simulink model "Path_planner_with_controller_localization"  (R2017b)
settings: Solver=FixedStepDiscrete  StartTime=0.0  StopTime=t  FixedStep=dt  RelTol=1e-3
values from neighbouring files (symbols this model uses):
  d = 0.15    [extendedKalman.m]    (also in extendedKalmanFilter.m; plant.m = 0.24; runV3.m; runpathfollower.m)
  dt = 0.1    [extendedKalmanFilter.m]    (also in matlab.mat; runV3.m; rungen.m; runpathfollower.m)
  k1 = 8    [runpathfollower.m]    (also in runpathplanner.m = 1)
  k2 = 1    [runpathfollower.m]    (also in runpathplanner.m)
  pl = 4    [runpathfollower.m]    (also in runpathplanner.m = 10)
  pr = 1    [runpathfollower.m]
  pthetai = 45*pi/180    (= 0.785398163397)    [runpathfollower.m]    (also in runpathplanner.m)
  pxi = 2    [runpathfollower.m]    (also in runpathplanner.m = 0)
  pyi = 2    [runpathfollower.m]    (also in runpathplanner.m)
  velocity = 0.3    [runpathfollower.m]    (also in runpathplanner.m)
  xi0 = [0 0 0 0 0 0 0 0]    [matlab.mat]    (also in runV3.m = [0 0 0 0 0 0 0 0]'; runpathfollower.m = [xi,yi,0,0,0,0,theta_mi,0]'; runpathplanner.m = [xi,yi,0,0,0,0,theta_mi,0]')
libraries: simulink x10
settings Model: Creator=nisha  LastModifiedBy=nisha

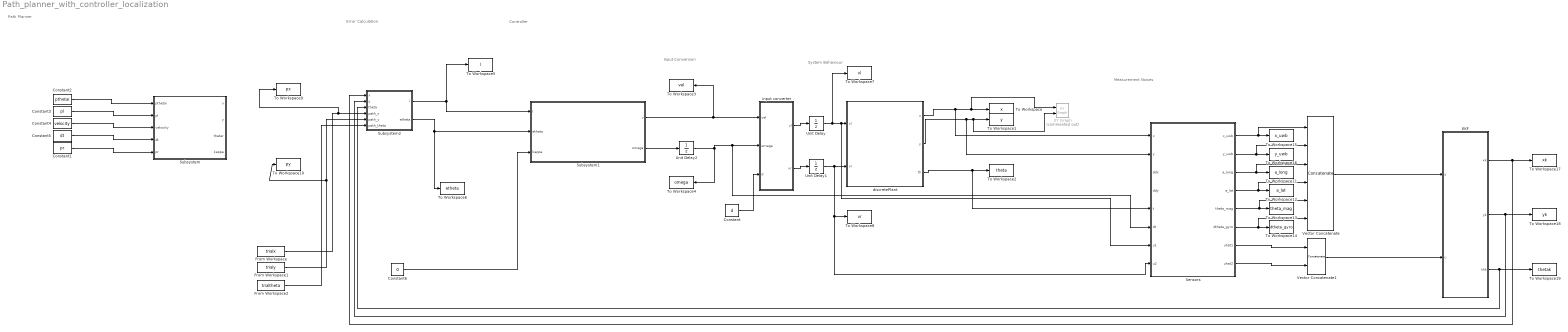
== system Path_planner_with_controller_localization ==
  note: Controller
  note: Error Calculation
  note: Measurement Noises
  note: System Behaviour
  note: Input Conversion
  note: Path Planner
  Constant : Constant  Value=d
  Constant1 : Constant  Value=pr
  Constant2 : Constant  Value=pthetai
  Constant3 : Constant  Value=pl
  Constant4 : Constant  Value=velocity
  Constant5 : Constant  Value=dt
  Constant6 : Constant  Value=0
  EKF : Subsystem
  From Workspace : FromWorkspace  VariableName=trialx
  From Workspace1 : FromWorkspace  VariableName=trialy
  From Workspace2 : FromWorkspace  VariableName=trialtheta
  Sensors : Subsystem  Description=dfg
  Subsystem : Subsystem
  Subsystem1 : Subsystem
  Subsystem2 : Subsystem
  To Workspace : ToWorkspace  VariableName=x  SampleTime=-1
  To Workspace1 : ToWorkspace  VariableName=y  SampleTime=-1
  To Workspace10 : ToWorkspace  VariableName=py  SampleTime=-1
  To Workspace11 : ToWorkspace  VariableName=a_long  SampleTime=-1
  To Workspace12 : ToWorkspace  VariableName=a_lat  SampleTime=-1
  To Workspace13 : ToWorkspace  VariableName=theta_mag  SampleTime=-1
  To Workspace14 : ToWorkspace  VariableName=dtheta_gyro  SampleTime=-1
  To Workspace15 : ToWorkspace  VariableName=x_uwb  SampleTime=-1
  To Workspace16 : ToWorkspace  VariableName=y_uwb  SampleTime=-1
  To Workspace17 : ToWorkspace  VariableName=xk  SampleTime=-1
  To Workspace18 : ToWorkspace  VariableName=yk  SampleTime=-1
  To Workspace19 : ToWorkspace  VariableName=thetak  SampleTime=-1
  To Workspace2 : ToWorkspace  VariableName=theta  SampleTime=-1
  To Workspace3 : ToWorkspace  VariableName=vel  SampleTime=-1
  To Workspace4 : ToWorkspace  VariableName=omega  SampleTime=-1
  To Workspace5 : ToWorkspace  VariableName=l  SampleTime=-1
  To Workspace6 : ToWorkspace  VariableName=etheta  SampleTime=-1
  To Workspace7 : ToWorkspace  VariableName=vl  SampleTime=-1
  To Workspace8 : ToWorkspace  VariableName=vr  SampleTime=-1
  To Workspace9 : ToWorkspace  VariableName=px  SampleTime=-1
  Unit Delay : UnitDelay  SampleTime=-1
  Unit Delay1 : UnitDelay  SampleTime=-1
  Unit Delay2 : UnitDelay  SampleTime=-1
  Vector Concatenate : Concatenate  NumInputs=6
  Vector Concatenate1 : Concatenate
  XY Graph : simulink/Sinks/XY Graph  Commented=on  xmin=0  xmax=10  ymin=2  ymax=12  st=-1
  discretePlant : Subsystem
  input converter : MATLAB Function  TreatAsAtomicUnit=on
  wires:
  Constant4/1 -> Subsystem/3(velocity)
  Constant3/1 -> Subsystem/2(pl)
  Constant2/1 -> Subsystem/1(pthetai)
  Constant5/1 -> Subsystem/4(dt)
  discretePlant/3(th) -> Sensors/5(t), To Workspace2/1
  Subsystem2/1(l) -> Subsystem1/1(l), To Workspace5/1
  Subsystem2/2(etheta) -> To Workspace6/1, Subsystem1/2(etheta)
  input converter/2(vr) -> Unit Delay1/1
  discretePlant/1(x) -> Sensors/1(x), XY Graph/1, To Workspace/1
  Constant/1 -> input converter/3(d)
  Subsystem1/1(v) -> To Workspace3/1, input converter/1(vel)
  Unit Delay/1 -> To Workspace7/1, Sensors/7(u1), discretePlant/1(vl)
  discretePlant/2(y) -> Sensors/2(y), XY Graph/2, To Workspace1/1
  input converter/1(vl) -> Unit Delay/1
  Subsystem1/2(omega) -> Unit Delay2/1
  Constant1/1 -> Subsystem/5(pr)
  Sensors/6(dtheta_gyro) -> To Workspace14/1, Vector Concatenate/6
  Sensors/8(uhat2) -> Vector Concatenate1/2
  Vector Concatenate1/1 -> EKF/2(u)
  Sensors/7(uhat1) -> Vector Concatenate1/1
  Sensors/3(a_long) -> Vector Concatenate/3, To Workspace11/1
  Sensors/5(theta_mag) -> Vector Concatenate/5, To Workspace13/1
  EKF/1(xk) -> To Workspace17/1, Subsystem2/1(x)
  Sensors/4(a_lat) -> Vector Concatenate/4, To Workspace12/1
  Sensors/1("x_uwb ") -> Vector Concatenate/1, To Workspace15/1
  Vector Concatenate/1 -> EKF/1(y)
  Sensors/2(y_uwb) -> Vector Concatenate/2, To Workspace16/1
  Unit Delay1/1 -> To Workspace8/1, Sensors/8(u2), discretePlant/2(vr)
  EKF/2(yk) -> To Workspace18/1, Subsystem2/2(y)
  EKF/3(thk) -> To Workspace19/1, Subsystem2/3(theta)
  Unit Delay2/1 -> Sensors/6(dt), input converter/2(omega), To Workspace4/1
  Constant6/1 -> Subsystem1/3(kappa)
  From Workspace/1 -> To Workspace9/1, Subsystem2/4(path_x)
  From Workspace1/1 -> To Workspace10/1, Subsystem2/5(path_y)
  From Workspace2/1 -> Subsystem2/6(path_theta)

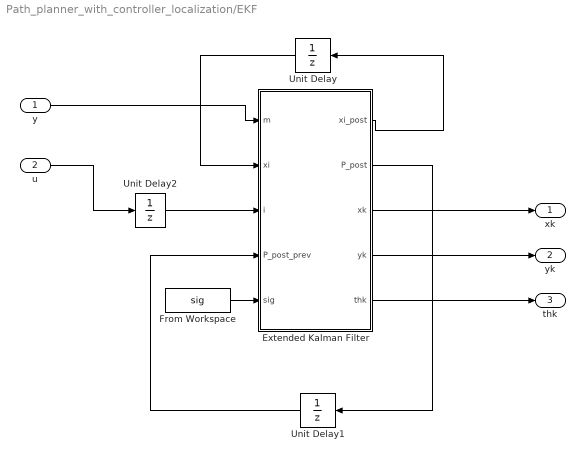
== system Path_planner_with_controller_localization/EKF ==
  y : Inport
  u : Inport  Port=2
  Extended Kalman Filter : MATLAB Function  TreatAsAtomicUnit=on
  From Workspace : FromWorkspace  VariableName=sig  SampleTime=0
  Unit Delay : UnitDelay  InitialCondition=xi0  SampleTime=-1
  Unit Delay1 : UnitDelay  InitialCondition=zeros(8,8)  SampleTime=-1
  Unit Delay2 : UnitDelay  InitialCondition=[0;0]  SampleTime=-1
  xk : Outport
  yk : Outport  Port=2
  thk : Outport  Port=3
  wires:
  Extended Kalman Filter/1(xi_post) -> Unit Delay/1
  y/1 -> Extended Kalman Filter/1(m)
  u/1 -> Unit Delay2/1
  Unit Delay2/1 -> Extended Kalman Filter/3(i)
  Unit Delay/1 -> Extended Kalman Filter/2(xi)
  Extended Kalman Filter/2(P_post) -> Unit Delay1/1
  Unit Delay1/1 -> Extended Kalman Filter/4(P_post_prev)
  Extended Kalman Filter/3(xk) -> xk/1
  Extended Kalman Filter/4(yk) -> yk/1
  From Workspace/1 -> Extended Kalman Filter/5(sig)
  Extended Kalman Filter/5(thk) -> thk/1

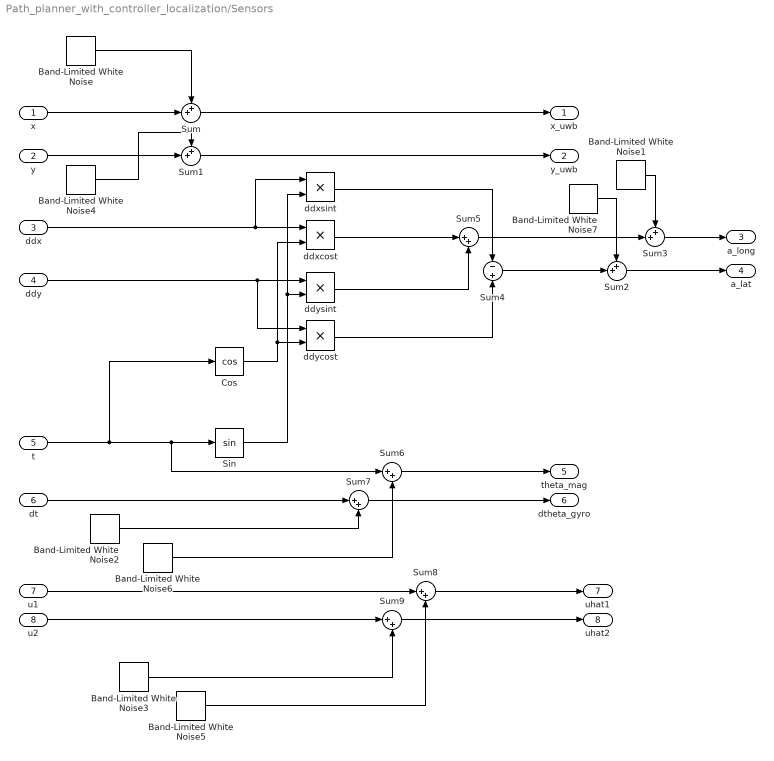
== system Path_planner_with_controller_localization/Sensors ==
  x : Inport
  y : Inport  Port=2
  ddx : Inport  Port=3
  ddy : Inport  Port=4
  t : Inport  Port=5
  dt : Inport  Port=6
  u1 : Inport  Port=7
  u2 : Inport  Port=8
  Band-Limited White Noise : simulink/Sources/Band-Limited White Noise  Cov=noiseUWB  Ts=dt  seed=[23341]
  Band-Limited White Noise1 : simulink/Sources/Band-Limited White Noise  Cov=noiseAcc  Ts=dt  seed=[23341]
  Band-Limited White Noise2 : simulink/Sources/Band-Limited White Noise  Cov=noiseGyro  Ts=dt  seed=[23341]
  Band-Limited White Noise3 : simulink/Sources/Band-Limited White Noise  Cov=noiseIn  Ts=dt  seed=[23341]
  Band-Limited White Noise4 : simulink/Sources/Band-Limited White Noise  Cov=noiseUWB  Ts=dt  seed=[23241]
  Band-Limited White Noise5 : simulink/Sources/Band-Limited White Noise  Cov=noiseIn  Ts=dt  seed=[23341]
  Band-Limited White Noise6 : simulink/Sources/Band-Limited White Noise  Cov=noiseMag  Ts=dt  seed=[23341]
  Band-Limited White Noise7 : simulink/Sources/Band-Limited White Noise  Cov=noiseAcc  Ts=dt  seed=[23341]
  Cos : Trigonometry  Operator=cos
  Sin : Trigonometry
  Sum{,1..3} (4 alike) : Sum  Inputs=++|
  Sum4 : Sum  Inputs=-|+
  Sum{5..9} (5 alike) : Sum  Inputs=|++
  ddxcost : Product
  ddxsint : Product
  ddycost : Product
  ddysint : Product
  "x_uwb " : Outport
  y_uwb : Outport  Port=2
  a_long : Outport  Port=3
  a_lat : Outport  Port=4
  theta_mag : Outport  Port=5
  dtheta_gyro : Outport  Port=6
  uhat1 : Outport  Port=7
  uhat2 : Outport  Port=8
  wires:
  x/1 -> Sum/2
  y/1 -> Sum1/2
  Band-Limited White Noise/1 -> Sum/1
  Sum/1 -> "x_uwb "/1
  Sum1/1 -> y_uwb/1
  Band-Limited White Noise1/1 -> Sum3/1
  t/1 -> Sum6/1, Sin/1, Cos/1
  ddx/1 -> ddxcost/1, ddxsint/1
  Cos/1 -> ddxcost/2, ddycost/2
  Sin/1 -> ddxsint/2, ddysint/2
  ddy/1 -> ddycost/1, ddysint/1
  Sum5/1 -> Sum3/2
  Sum4/1 -> Sum2/2
  ddxcost/1 -> Sum5/1
  ddysint/1 -> Sum5/2
  ddxsint/1 -> Sum4/1
  ddycost/1 -> Sum4/2
  Sum6/1 -> theta_mag/1
  dt/1 -> Sum7/1
  Sum7/1 -> dtheta_gyro/1
  Band-Limited White Noise2/1 -> Sum7/2
  Sum3/1 -> a_long/1
  Sum2/1 -> a_lat/1
  Band-Limited White Noise3/1 -> Sum9/2
  Sum9/1 -> uhat2/1
  u2/1 -> Sum9/1
  Sum8/1 -> uhat1/1
  u1/1 -> Sum8/1
  Band-Limited White Noise4/1 -> Sum1/1
  Band-Limited White Noise5/1 -> Sum8/2
  Band-Limited White Noise6/1 -> Sum6/2
  Band-Limited White Noise7/1 -> Sum2/1

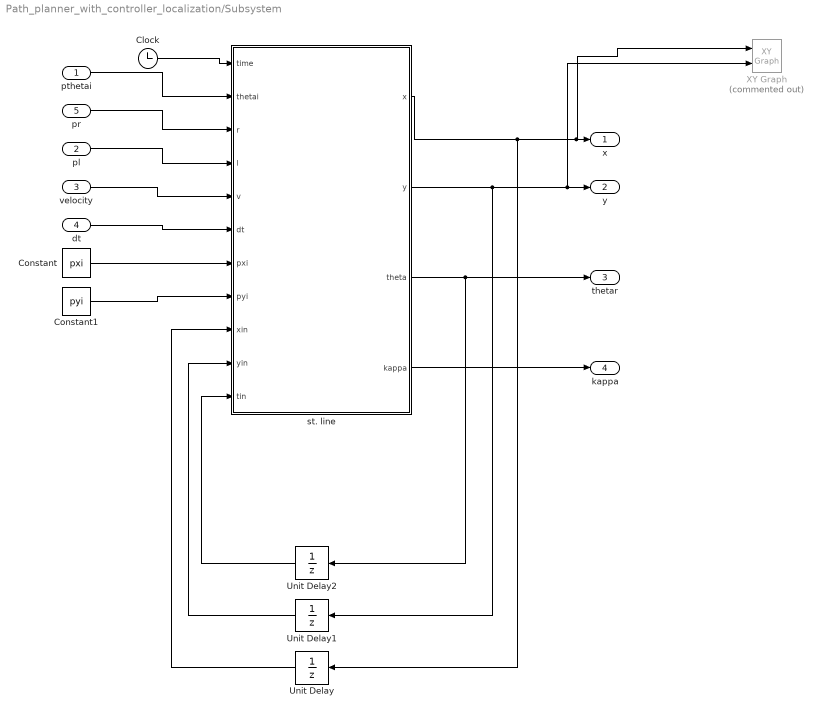
== system Path_planner_with_controller_localization/Subsystem ==
  pthetai : Inport
  pl : Inport  Port=2
  velocity : Inport  Port=3
  dt : Inport  Port=4
  pr : Inport  Port=5
  Clock : Clock
  Constant : Constant  Value=pxi
  Constant1 : Constant  Value=pyi
  Unit Delay : UnitDelay  InitialCondition=pxi  SampleTime=-1
  Unit Delay1 : UnitDelay  InitialCondition=pyi  SampleTime=-1
  Unit Delay2 : UnitDelay  InitialCondition=pthetai  SampleTime=-1
  XY Graph : simulink/Sinks/XY Graph  Commented=on  xmin=0  xmax=10  ymin=2  ymax=12  st=-1
  st. line : MATLAB Function  TreatAsAtomicUnit=on
  x : Outport
  y : Outport  Port=2
  thetar : Outport  Port=3
  kappa : Outport  Port=4
  wires:
  pthetai/1 -> st. line/2(thetai)
  pl/1 -> st. line/4(l)
  velocity/1 -> st. line/5(v)
  st. line/2(y) -> Unit Delay1/1, XY Graph/2, y/1
  dt/1 -> st. line/6(dt)
  Unit Delay/1 -> st. line/9(xin)
  Unit Delay1/1 -> st. line/10(yin)
  Constant/1 -> st. line/7(pxi)
  Constant1/1 -> st. line/8(pyi)
  Clock/1 -> st. line/1(time)
  st. line/3(theta) -> Unit Delay2/1, thetar/1
  pr/1 -> st. line/3(r)
  Unit Delay2/1 -> st. line/11(tin)
  st. line/1(x) -> Unit Delay/1, XY Graph/1, x/1
  st. line/4(kappa) -> kappa/1

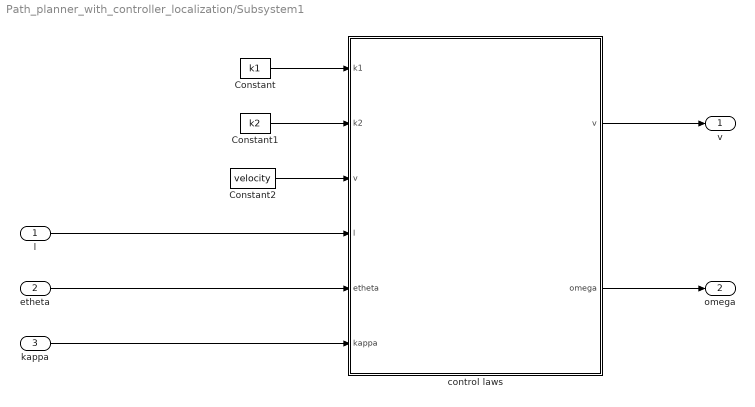
== system Path_planner_with_controller_localization/Subsystem1 ==
  l : Inport
  etheta : Inport  Port=2
  kappa : Inport  Port=3
  Constant : Constant  Value=k1
  Constant1 : Constant  Value=k2
  Constant2 : Constant  Value=velocity
  control laws : MATLAB Function  TreatAsAtomicUnit=on
  v : Outport
  omega : Outport  Port=2
  wires:
  Constant/1 -> control laws/1(k1)
  Constant1/1 -> control laws/2(k2)
  Constant2/1 -> control laws/3("v ")
  l/1 -> control laws/4(l)
  etheta/1 -> control laws/5(etheta)
  kappa/1 -> control laws/6(kappa)
  control laws/1(v) -> v/1
  control laws/2(omega) -> omega/1

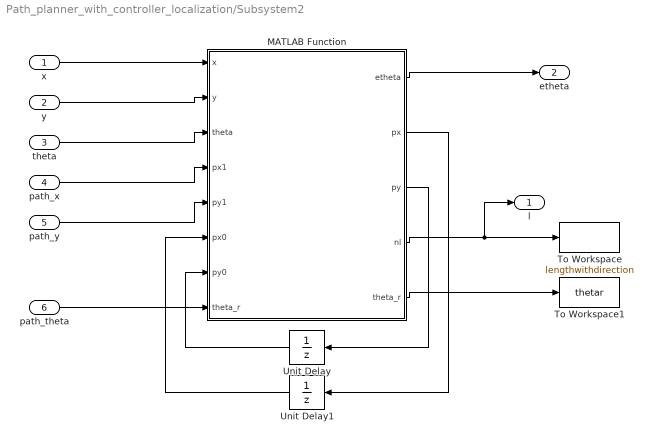
== system Path_planner_with_controller_localization/Subsystem2 ==
  x : Inport
  y : Inport  Port=2
  theta : Inport  Port=3
  path_x : Inport  Port=4
  path_y : Inport  Port=5
  path_theta : Inport  Port=6
  MATLAB Function : MATLAB Function  TreatAsAtomicUnit=on
  To Workspace : ToWorkspace  VariableName=lengthwithdirection  SampleTime=-1
  To Workspace1 : ToWorkspace  VariableName=thetar  SampleTime=-1
  Unit Delay : UnitDelay  InitialCondition=pyi  SampleTime=-1
  Unit Delay1 : UnitDelay  InitialCondition=pxi  SampleTime=-1
  l : Outport
  etheta : Outport  Port=2
  wires:
  x/1 -> MATLAB Function/1(x)
  y/1 -> MATLAB Function/2(y)
  path_x/1 -> MATLAB Function/4(px1)
  theta/1 -> MATLAB Function/3(theta)
  MATLAB Function/1(etheta) -> etheta/1
  MATLAB Function/4(nl) -> To Workspace/1, l/1
  MATLAB Function/2(px) -> Unit Delay1/1
  MATLAB Function/3(py) -> Unit Delay/1
  path_y/1 -> MATLAB Function/5(py1)
  Unit Delay/1 -> MATLAB Function/7(py0)
  Unit Delay1/1 -> MATLAB Function/6(px0)
  MATLAB Function/5(theta_r) -> To Workspace1/1
  path_theta/1 -> MATLAB Function/8("theta_r ")

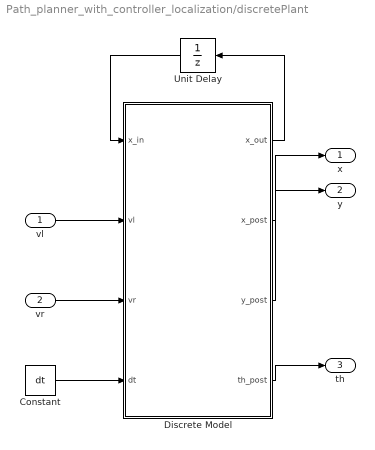
== system Path_planner_with_controller_localization/discretePlant ==
  vl : Inport
  vr : Inport  Port=2
  Constant : Constant  Value=dt
  Discrete Model : MATLAB Function  TreatAsAtomicUnit=on
  Unit Delay : UnitDelay  InitialCondition=xi0  SampleTime=-1
  x : Outport
  y : Outport  Port=2
  th : Outport  Port=3
  wires:
  vl/1 -> Discrete Model/2(vl)
  Discrete Model/1(x_out) -> Unit Delay/1
  Unit Delay/1 -> Discrete Model/1(x_in)
  vr/1 -> Discrete Model/3(vr)
  Discrete Model/2(x_post) -> x/1
  Discrete Model/3(y_post) -> y/1
  Discrete Model/4(th_post) -> th/1
  Constant/1 -> Discrete Model/4(dt)

== matlab function Path_planner_with_controller_localization/Subsystem1/control laws ==
  data: k1 input; v output; k2 input; v input; l input; etheta input; kappa input; omega output
function [v,omega] = fcn(k1, k2, v, l, etheta, kappa)
omega= kappa*cos(etheta)*v/(1-kappa*l)-k1*l*v*sin(etheta)/etheta-k2*etheta;
t=1;

== matlab function Path_planner_with_controller_localization/Subsystem/st. line ==
  data: time input; x output; y output; thetai input; r input; l input; v input; dt input; pxi input; pyi input; xin input; yin input; theta output; tin input; kappa output
function [x,y,theta,kappa] = fcn(time,thetai,r,l,v,dt,pxi,pyi,xin,yin,tin)

dl=dt*v;
dtt=dl/r;
if time<l/v
   x=xin+dl*cos(thetai); 
   y=yin+dl*sin(thetai);
   theta=atan((y-yin)/(x-xin));
   kappa=0;
elseif (time>l/v-dt) && ((tin-thetai)<pi) && (time<l/v+r*10)
   theta=tin+dtt;
   x=xin+dl*cos(theta); 
   y=yin+dl*sin(theta);
   kappa=1;
%    theta=atan((y-yin)/(x-xin));
else
    theta=thetai+pi;
    x=xin+dl*cos(tin);
    y=yin+dl*sin(tin);
    kappa=0;
end
end

== matlab function Path_planner_with_controller_localization/Subsystem2/MATLAB Function ==
  data: x input; y input; theta input; px1 input; etheta output; py1 input; px output; py output; px0 input; py0 input; nl output; theta_r output; theta_r input
function [ etheta,px,py,nl,theta_r] = fcn(x,y,theta,px1,py1,px0,py0,theta_r)
v=[px1-px0,py1-py0];
w=[x-px0,y-py0];
px=px1; py=py1;
% theta_r=atan(v(2)/v(1));

rot=[cos(theta_r) sin(theta_r)
    -sin(theta_r) cos(theta_r)];
length=rot*w';
nl=dot(length,[0; 1]);
etheta=theta-theta_r;

== matlab function Path_planner_with_controller_localization/discretePlant/Discrete Model ==
  data: x_in input; x_out output; vl input; vr input; x_post output; y_post output; th_post output; dt input
function [x_out,x_post,y_post,th_post]         = fcn(x_in,vl, vr,dt)

d=0.15;
x=x_in(1); y=x_in(2); dx=x_in(3);dy=x_in(4);ddx=x_in(5);ddy=x_in(6); phi=x_in(7); dphi=x_in(8);
th=phi+0.5*dphi*dt;
x_out = ...
[x + dx*dt + ddx*dt^2/2
 y + dy*dt + ddy*dt^2/2
 (vl+vr)/2*cos(th)+ddx*dt
 (vl+vr)/2*sin(th)+ddy*dt
 ddx
 ddy
 phi + dphi*dt
 (vr-vl)/d];

x_post=x_out(1); y_post=x_out(2); th_post=x_out(7);
end

== matlab function Path_planner_with_controller_localization/input converter ==
  data: vel input; vl output; omega input; d input; vr output
function [vl, vr] = fcn(vel, omega,d)
vr=vel +d/2*omega;
vl=vel -d/2*omega;
end

== matlab function Path_planner_with_controller_localization/EKF/Extended Kalman Filter ==
  data: m input; xi input; i input; P_post_prev input; xi_post output; P_post output; xk output; yk output; sig input; thk output
function [xi_post,P_post,xk,yk, thk] = fcn(m,xi,i,P_post_prev,sig)
%% Prediction

d=0.15; dt=0.1;
x=xi(1); y=xi(2); dx=xi(3); dy=xi(4); ddx=xi(5); ddy=xi(6); phi=xi(7); dphi=xi(8);
th=phi+0.5*dphi*dt;
vl=i(1); vr=i(2);
xi_prio = ...
            [ x + dx*dt + ddx*dt^2/2
              y + dy*dt + ddy*dt^2/2
             (vl+vr)/2*cos(th)+ddx*dt
             (vl+vr)/2*sin(th)+ddy*dt
             ddx
             ddy
             phi + dphi*dt
             (vr-vl)/d               ];

A = ...
        [ 1, 0, dt,  0, dt^2/2,      0,                              0,                             0
          0, 1,  0, dt,      0, dt^2/2,                              0,                             0
          0, 0,  0,  0,     dt,      0,         -sin(th)*(vl/2 + vr/2), -(dt*sin(th)*(vl/2 + vr/2))/2
          0, 0,  0,  0,      0,     dt,          cos(th)*(vl/2 + vr/2),  (dt*cos(th)*(vl/2 + vr/2))/2
          0, 0,  0,  0,      1,      0,                              0,                             0
          0, 0,  0,  0,      0,      1,                              0,                             0
          0, 0,  0,  0,      0,      0,                              1,                             dt
          0, 0,  0,  0,      0,      0,                              0,                             0];

V= ...
    [         0,         0
              0,         0
      cos(th)/2, cos(th)/2
      sin(th)/2, sin(th)/2
              0,         0
              0,         0
              0,         0
           -1/d,       1/d];
sigx=sig(1);sigy=sig(2);sigdx=sig(3);sigdy=sig(4);sigddx=sig(5);sigddy=sig(6);sigphi=sig(7);
sigdphi=sig(8);sigvl=sig(9);sigvr=sig(9);

Q = diag([sigx,sigy,sigdx,sigdy,sigddx,sigddy,sigphi,sigdphi]);
M=diag([sigvl,sigvr]);
P_prio = A*P_post_prev*A'+Q + V*M*V';

%% Update
zhat = [1    0   0   0   0           0           0   0
        0    1   0   0   0           0           0   0
        0    0   0   0   cosd(phi)    sind(phi)    0   0
        0    0   0   0   -sind(phi)   cosd(phi)    0   0
        0    0   0   0   0           0           1   0
        0    0   0   0   0           0           0   1]*xi_prio;
C =  [1, 0, 0, 0,         0,        0,                             0, 0;
      0, 1, 0, 0,         0,        0,                             0, 0;
      0, 0, 0, 0,  cosd(phi), sind(phi),   ddy*cosd(phi) - ddx*sind(phi), 0;
      0, 0, 0, 0, -sind(phi), cosd(phi), - ddx*cosd(phi) - ddy*sind(phi), 0;
      0, 0, 0, 0,         0,        0,                             1, 0;
      0, 0, 0, 0,         0,        0,                             0, 1];
R = diag([10,10, 0.01/dt, 0.01/dt, 0.001/dt, 0.001/dt]);
K = P_prio*C'/(C*P_prio*C'+R);


% Update states and covariance matrix
xi_post = xi_prio + K*(m-zhat);
P_post = (eye(size(P_prio,1))-K*C)*P_prio; %*(eye(size(P_prio,1))-K*C)'+K*R*K';
xk=xi_post(1); yk=xi_post(2); thk=xi_post(7);
